simulink model "IEEE14_case"  (R2024b)
settings: Solver=FixedStepAuto  StartTime=0  StopTime=2  FixedStep=1e-7  RelTol=1e-3
values from neighbouring files (symbols this model uses):
  GFL_15_Bva = 0.009    [IEEE14_parameters.m]
  GFL_15_C_bus_pu = 7.179419    [IEEE14_parameters.m]
  GFL_15_f0 = 60    [IEEE14_parameters.m]
  GFL_15_I_id = 691.26967    [IEEE14_parameters.m]
  GFL_15_I_iq = 691.26967    [IEEE14_parameters.m]
  GFL_15_I_od = 45.2207    [IEEE14_parameters.m]
  GFL_15_I_oq = 45.2207    [IEEE14_parameters.m]
  GFL_15_I_pll = 0.78    [IEEE14_parameters.m]
  GFL_15_Kdi = 0.09    [IEEE14_parameters.m]
  GFL_15_Kdo = 0.9    [IEEE14_parameters.m]
  GFL_15_Kqi = 0.09    [IEEE14_parameters.m]
  GFL_15_Kqo = 0.9    [IEEE14_parameters.m]
  GFL_15_Lg_pu = 0.631447    [IEEE14_parameters.m]
  GFL_15_mode = 1    [IEEE14_parameters.m]
  GFL_15_P_id = 3.7166    [IEEE14_parameters.m]
  GFL_15_P_iq = 3.7166    [IEEE14_parameters.m]
  GFL_15_P_od = 0.4798    [IEEE14_parameters.m]
  GFL_15_P_oq = 0.4798    [IEEE14_parameters.m]
  GFL_15_P_pll = 290.42    [IEEE14_parameters.m]
  GFL_15_Qe_ref = 0.2    [IEEE14_parameters.m]
  GFL_15_Rg_pu = 0.024016    [IEEE14_parameters.m]
  GFL_15_Sbase = 1.000000e+4    (= 10000)    [IEEE14_parameters.m]
  GFL_15_Tdi = 0.01    [IEEE14_parameters.m]
  GFL_15_Tdo = 0.2    [IEEE14_parameters.m]
  GFL_15_Tqi = 0.01    [IEEE14_parameters.m]
  GFL_15_Tqo = 0.2    [IEEE14_parameters.m]
  GFL_15_Vbase = 380    [IEEE14_parameters.m]
  GFL_15_Vdc_ref = 1.011475    [IEEE14_parameters.m]
  GFL_15_Vdcbase = 700    [IEEE14_parameters.m]
  GFL_15_vq_ref = 0    [IEEE14_parameters.m]
  GFL_16_Bva = 0.002    [IEEE14_parameters.m]
  GFL_16_C_bus_pu = 7.179419    [IEEE14_parameters.m]
  GFL_16_f0 = 60    [IEEE14_parameters.m]
  GFL_16_I_id = 691.26967    [IEEE14_parameters.m]
  GFL_16_I_iq = 691.26967    [IEEE14_parameters.m]
  GFL_16_I_od = 45.2207    [IEEE14_parameters.m]
  GFL_16_I_oq = 45.2207    [IEEE14_parameters.m]
  GFL_16_I_pll = 0.78    [IEEE14_parameters.m]
  GFL_16_Kdi = 0.05    [IEEE14_parameters.m]
  GFL_16_Kdo = 0.5    [IEEE14_parameters.m]
  GFL_16_Kqi = 0.05    [IEEE14_parameters.m]
  GFL_16_Kqo = 0.5    [IEEE14_parameters.m]
  GFL_16_Lg_pu = 0.631447    [IEEE14_parameters.m]
  GFL_16_mode = 1    [IEEE14_parameters.m]
  GFL_16_P_id = 3.7166    [IEEE14_parameters.m]
  GFL_16_P_iq = 3.7166    [IEEE14_parameters.m]
  GFL_16_P_od = 0.4798    [IEEE14_parameters.m]
  GFL_16_P_oq = 0.4798    [IEEE14_parameters.m]
  GFL_16_P_pll = 290.42    [IEEE14_parameters.m]
  GFL_16_Qe_ref = 0.2    [IEEE14_parameters.m]
  GFL_16_Rg_pu = 0.024016    [IEEE14_parameters.m]
  GFL_16_Sbase = 1.000000e+4    (= 10000)    [IEEE14_parameters.m]
  GFL_16_Tdi = 0.01    [IEEE14_parameters.m]
  GFL_16_Tdo = 0.2    [IEEE14_parameters.m]
  GFL_16_Tqi = 0.01    [IEEE14_parameters.m]
  GFL_16_Tqo = 0.2    [IEEE14_parameters.m]
  GFL_16_Vbase = 380    [IEEE14_parameters.m]
  GFL_16_Vdc_ref = 1.01144    [IEEE14_parameters.m]
  GFL_16_Vdcbase = 700    [IEEE14_parameters.m]
  GFL_16_vq_ref = 0    [IEEE14_parameters.m]
  GFL_17_Bva = 0.002    [IEEE14_parameters.m]
  GFL_17_C_bus_pu = 7.179419    [IEEE14_parameters.m]
  GFL_17_f0 = 60    [IEEE14_parameters.m]
  GFL_17_I_id = 691.26967    [IEEE14_parameters.m]
  GFL_17_I_iq = 691.26967    [IEEE14_parameters.m]
  GFL_17_I_od = 45.2207    [IEEE14_parameters.m]
  GFL_17_I_oq = 45.2207    [IEEE14_parameters.m]
  GFL_17_I_pll = 0.78    [IEEE14_parameters.m]
  GFL_17_Kdi = 0.05    [IEEE14_parameters.m]
  GFL_17_Kdo = 0.5    [IEEE14_parameters.m]
  GFL_17_Kqi = 0.05    [IEEE14_parameters.m]
  GFL_17_Kqo = 0.5    [IEEE14_parameters.m]
  GFL_17_Lg_pu = 0.631447    [IEEE14_parameters.m]
  GFL_17_mode = 1    [IEEE14_parameters.m]
  GFL_17_P_id = 3.7166    [IEEE14_parameters.m]
  GFL_17_P_iq = 3.7166    [IEEE14_parameters.m]
  GFL_17_P_od = 0.4798    [IEEE14_parameters.m]
  GFL_17_P_oq = 0.4798    [IEEE14_parameters.m]
  GFL_17_P_pll = 290.42    [IEEE14_parameters.m]
  GFL_17_Qe_ref = 0.2    [IEEE14_parameters.m]
  GFL_17_Rg_pu = 0.024016    [IEEE14_parameters.m]
  GFL_17_Sbase = 1.000000e+4    (= 10000)    [IEEE14_parameters.m]
  GFL_17_Tdi = 0.01    [IEEE14_parameters.m]
  GFL_17_Tdo = 0.2    [IEEE14_parameters.m]
  GFL_17_Tqi = 0.01    [IEEE14_parameters.m]
  GFL_17_Tqo = 0.2    [IEEE14_parameters.m]
  GFL_17_Vbase = 380    [IEEE14_parameters.m]
  GFL_17_Vdc_ref = 1.011632    [IEEE14_parameters.m]
  GFL_17_Vdcbase = 700    [IEEE14_parameters.m]
  GFL_17_vq_ref = 0    [IEEE14_parameters.m]
  GFL_18_Bva = 0.002    [IEEE14_parameters.m]
  GFL_18_C_bus_pu = 7.179419    [IEEE14_parameters.m]
  GFL_18_f0 = 60    [IEEE14_parameters.m]
  GFL_18_I_id = 691.26967    [IEEE14_parameters.m]
  GFL_18_I_iq = 691.26967    [IEEE14_parameters.m]
  GFL_18_I_od = 45.2207    [IEEE14_parameters.m]
  GFL_18_I_oq = 45.2207    [IEEE14_parameters.m]
  GFL_18_I_pll = 0.78    [IEEE14_parameters.m]
  GFL_18_Kdi = 0.05    [IEEE14_parameters.m]
  GFL_18_Kdo = 0.5    [IEEE14_parameters.m]
  GFL_18_Kqi = 0.05    [IEEE14_parameters.m]
  GFL_18_Kqo = 0.5    [IEEE14_parameters.m]
  GFL_18_Lg_pu = 0.631447    [IEEE14_parameters.m]
  GFL_18_mode = 1    [IEEE14_parameters.m]
  GFL_18_P_id = 3.7166    [IEEE14_parameters.m]
  GFL_18_P_iq = 3.7166    [IEEE14_parameters.m]
  GFL_18_P_od = 0.4798    [IEEE14_parameters.m]
  GFL_18_P_oq = 0.4798    [IEEE14_parameters.m]
  GFL_18_P_pll = 290.42    [IEEE14_parameters.m]
  GFL_18_Qe_ref = 0.2    [IEEE14_parameters.m]
  GFL_18_Rg_pu = 0.024016    [IEEE14_parameters.m]
  GFL_18_Sbase = 1.000000e+4    (= 10000)    [IEEE14_parameters.m]
  GFL_18_Tdi = 0.01    [IEEE14_parameters.m]
  GFL_18_Tdo = 0.2    [IEEE14_parameters.m]
  GFL_18_Tqi = 0.01    [IEEE14_parameters.m]
  GFL_18_Tqo = 0.2    [IEEE14_parameters.m]
  GFL_18_Vbase = 380    [IEEE14_parameters.m]
  GFL_18_Vdc_ref = 1.011572    [IEEE14_parameters.m]
  GFL_18_Vdcbase = 700    [IEEE14_parameters.m]
  GFL_18_vq_ref = 0    [IEEE14_parameters.m]
  ... (+180 more)
(part 10 of 25)

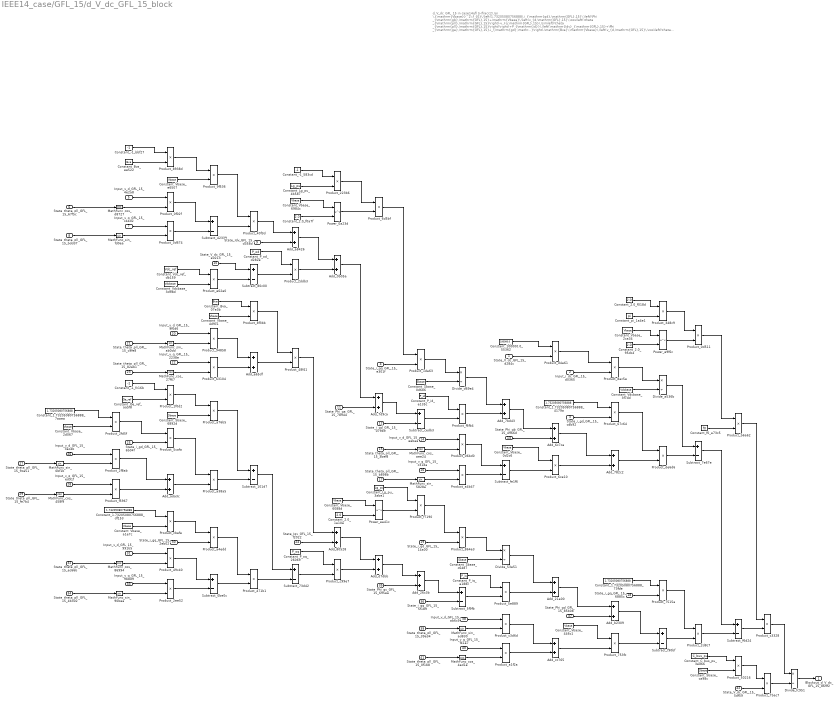
== system IEEE14_case/GFL_15/d_V_dc_GFL_15_block ==
  note: d_V_dc_GFL_15 in case14gfl
      | $-\frac{2\,\pi \,{\mathrm{Vbase}}^2\,f_{0}\,\left(1.73205080756888\,i_{\mathrm{gd},\mathrm{GFL},15}\,\left(\Phi _{\mathrm{gb},\mathrm{GFL},15}+\mathrm{Vbase}\,\left(v_{d,\mathrm{GFL},15}\,\cos\left(\theta _{\mathrm{pll},\mathrm{GFL},15}\right)-v_{q,\mathrm{GFL},15}\,\sin\left(\theta _{\mathrm{pll},\mathrm{GFL},15}\right)\right)+P_{\mathrm{id}}\,\left(\mathrm{Idv}_{\mathrm{GFL},15}+\Phi _{\mathrm{ga},\mathrm{GFL},15}-i_{\mathrm{gd},\mathrm{GFL},15}+P_{\mathrm{od}}\,\left(V_{\mathrm{dc},\mathrm{GFL},15}-\mathrm{Vdcbase}\,\mathrm{Vdc}_{\mathrm{ref}}\right)-\mathrm{Bva}\,\mathrm{Vbase}\,\left(v_{d,\mathrm{GFL},15}\,\cos\left(\theta _{\mathrm{pll},\mathrm{GFL},15}\right)-v_{q,\mathrm{GFL},15}\,\sin\left(\theta _{\mathrm{pll},\mathrm{GFL},15}\right)\right)\right)-\frac{\mathrm{Lg}_{\mathrm{pu}}\,{\mathrm{Vbase}}^2\,i_{\mathrm{gq},\mathrm{GFL},15}}{\mathrm{Sbase}}\right)+1.73205080756888\,i_{\mathrm{gq},\mathrm{GFL},15}\,\left(\Phi _{\mathrm{gd},\mathrm{GFL},15}-\mathrm{Vbase}\,\left(v_{q,\mathrm{GFL},15}\,\cos\left(\theta _{\mathrm{pll},\mathrm{GFL},15}\right)+v_{d,\mathrm{GFL},15}\,\sin\left(\theta _{\mathrm{pll},\mathrm{GFL},15}\right)\right)+P_{\mathrm{iq}}\,\left(\mathrm{Iqv}_{\mathrm{GFL},15}+\Phi _{\mathrm{gc},\mathrm{GFL},15}-i_{\mathrm{gq},\mathrm{GFL},15}-P_{\mathrm{oq}}\,\left(\mathrm{Qe}_{\mathrm{ref}}\,\mathrm{Sbase}+1.73205080756888\,\mathrm{Vbase}\,i_{\mathrm{gd},\mathrm{GFL},15}\,\left(v_{q,\mathrm{GFL},15}\,\cos\left(\theta _{\mathrm{pll},\mathrm{GFL},15}\right)+v_{d,\mathrm{GFL},15}\,\sin\left(\theta _{\mathrm{pll},\mathrm{GFL},15}\right)\right)+1.73205080756888\,\mathrm{Vbase}\,i_{\mathrm{gq},\mathrm{GFL},15}\,\left(v_{d,\mathrm{GFL},15}\,\cos\left(\theta _{\mathrm{pll},\mathrm{GFL},15}\right)-v_{q,\mathrm{GFL},15}\,\sin\left(\theta _{\mathrm{pll},\mathrm{GFL},15}\right)\right)\right)+\mathrm{Bva}\,\mathrm{Vbase}\,\left(v_{q,\mathrm{GFL},15}\,\cos\left(\theta _{\mathrm{pll},\mathrm{GFL},15}\right)+v_{d,\mathrm{GFL},15}\,\sin\left(\theta _{\mathrm{pll},\mathrm{GFL},15}\right)\right)\right)+\frac{\mathrm{Lg}_{\mathrm{pu}}\,{\mathrm{Vbase}}^2\,i_{\mathrm{gd},\mathrm{GFL},15}}{\mathrm{Sbase}}\right)-\frac{100000.0\,V_{\mathrm{dc},\mathrm{GFL},15}\,i_{\mathrm{dc},\mathrm{GFL},15}}{\mathrm{Vdcbase}}\right)}{C_{\mathrm{bus},\mathrm{pu}}\,\mathrm{Sbase}\,V_{\mathrm{dc},\mathrm{GFL},15}}$
      | Automatically generated on 2025-10-09 21:35:09 .
  State_V_dc_GFL_15_d284c : Inport
  Input_i_dc_GFL_15_d0365 : Inport  Port=2
  State_i_gd_GFL_15_cdb92 : Inport  Port=3
  State_i_gq_GFL_15_e301f : Inport  Port=4
  Input_v_d_GFL_15_4e2a8 : Inport  Port=5
  State_theta_pll_GFL_15_67f5c : Inport  Port=6
  Input_v_q_GFL_15_c44d2 : Inport  Port=7
  State_theta_pll_GFL_15_bdd37 : Inport  Port=8
  State_Idv_GFL_15_d358d : Inport  Port=9
  State_V_dc_GFL_15_e0213 : Inport  Port=10
  State_Phi_ga_GFL_15_78944 : Inport  Port=11
  State_i_gd_GFL_15_079b9 : Inport  Port=12
  State_Phi_gb_GFL_15_4966d : Inport  Port=13
  Input_v_d_GFL_15_eebae : Inport  Port=14
  State_theta_pll_GFL_15_3bef8 : Inport  Port=15
  Input_v_q_GFL_15_c31da : Inport  Port=16
  State_theta_pll_GFL_15_b898b : Inport  Port=17
  State_i_gq_GFL_15_6885c : Inport  Port=18
  State_i_gd_GFL_15_14a00 : Inport  Port=19
  Input_v_d_GFL_15_9f0d6 : Inport  Port=20
  State_theta_pll_GFL_15_c9fe8 : Inport  Port=21
  Input_v_q_GFL_15_2238e : Inport  Port=22
  State_theta_pll_GFL_15_82eb1 : Inport  Port=23
  State_Iqv_GFL_15_f2022 : Inport  Port=24
  State_i_gd_GFL_15_6b04f : Inport  Port=25
  Input_v_d_GFL_15_3ac4b : Inport  Port=26
  State_theta_pll_GFL_15_9ca51 : Inport  Port=27
  Input_v_q_GFL_15_ed91f : Inport  Port=28
  State_theta_pll_GFL_15_fe7b4 : Inport  Port=29
  State_i_gq_GFL_15_2eb02 : Inport  Port=30
  Input_v_d_GFL_15_991b5 : Inport  Port=31
  State_theta_pll_GFL_15_ec66b : Inport  Port=32
  Input_v_q_GFL_15_9b8d9 : Inport  Port=33
  State_theta_pll_GFL_15_4b302 : Inport  Port=34
  State_Phi_gc_GFL_15_695ea : Inport  Port=35
  State_i_gq_GFL_15_5f189 : Inport  Port=36
  State_Phi_gd_GFL_15_85b08 : Inport  Port=37
  Input_v_d_GFL_15_ab6c9 : Inport  Port=38
  State_theta_pll_GFL_15_39e34 : Inport  Port=39
  Input_v_q_GFL_15_f41a7 : Inport  Port=40
  State_theta_pll_GFL_15_0f1b8 : Inport  Port=41
  State_V_dc_GFL_15_5df59 : Inport  Port=42
  Add_0b05a : Sum
  Add_21a00 : Sum
  Add_26c3b : Sum
  Add_6c7ca : Sum
  Add_782c2 : Sum
  Add_7bd43 : Sum
  Add_7d9ca : Sum
  Add_80528 : Sum
  Add_a8426 : Sum
  Add_ada3c : Sum
  Add_b2309 : Sum
  Add_cc765 : Sum
  Add_d7dbb : Sum
  Add_e65df : Sum
  Constant_-1_583cd : Constant  Value=-1
  Constant_-1_bbf27 : Constant  Value=-1
  Constant_-1_fc16b : Constant  Value=-1
  Constant_1.73205080756888_4179a : Constant  Value=1.73205080756888
  Constant_1.73205080756888_73fde : Constant  Value=1.73205080756888
  Constant_1.73205080756888_7aaea : Constant  Value=1.73205080756888
  Constant_1.73205080756888_df153 : Constant  Value=1.73205080756888
  Constant_100000.0_55362 : Constant  Value=100000.0
  Constant_2.0_1a10a : Constant  Value=2.0
  Constant_2.0_95cb4 : Constant  Value=2.0
  Constant_2.0_f018d : Constant  Value=2.0
  Constant_2.0_f0a7f : Constant  Value=2.0
  Constant_Bva_07e3b : Constant  Value=Bva
  Constant_Bva_ee522 : Constant  Value=Bva
  Constant_C_bus_pu_3ed66 : Constant  Value=C_bus_pu
  Constant_Lg_pu_3abe1 : Constant  Value=Lg_pu
  Constant_Lg_pu_4b587 : Constant  Value=Lg_pu
  Constant_P_id_e135c : Constant  Value=P_id
  Constant_P_iq_a188c : Constant  Value=P_iq
  Constant_P_od_d282e : Constant  Value=P_od
  Constant_P_oq_26069 : Constant  Value=P_oq
  Constant_Qe_ref_aa5f8 : Constant  Value=Qe_ref
  Constant_Sbase_0d6b6 : Constant  Value=Sbase
  Constant_Sbase_6892d : Constant  Value=Sbase
  Constant_Sbase_c6487 : Constant  Value=Sbase
  Constant_Sbase_ca98c : Constant  Value=Sbase
  Constant_Vbase_0d2c6 : Constant  Value=Vbase
  Constant_Vbase_2ca34 : Constant  Value=Vbase
  Constant_Vbase_2d067 : Constant  Value=Vbase
  Constant_Vbase_446c1 : Constant  Value=Vbase
  Constant_Vbase_4d9c1 : Constant  Value=Vbase
  Constant_Vbase_6088d : Constant  Value=Vbase
  Constant_Vbase_6984c : Constant  Value=Vbase
  Constant_Vbase_a1e7c : Constant  Value=Vbase
  Constant_Vbase_e6507 : Constant  Value=Vbase
  Constant_Vdc_ref_db159 : Constant  Value=Vdc_ref
  Constant_Vdcbase_3d98d : Constant  Value=Vdcbase
  Constant_Vdcbase_3f7dd : Constant  Value=Vdcbase
  Constant_f0_a73c5 : Constant  Value=f0
  Constant_pi_1a4e1 : Constant  Value=pi
  Divide_53e51 : Product  Inputs=*/
  Divide_a536b : Product  Inputs=*/
  Divide_d69e4 : Product  Inputs=*/
  Divide_fc951 : Product  Inputs=*/
  MathFunc_cos_27f67 : Trigonometry  Operator=cos
  MathFunc_cos_458f9 : Trigonometry  Operator=cos
  MathFunc_cos_4ad1e : Trigonometry  Operator=cos
  MathFunc_cos_86994 : Trigonometry  Operator=cos
  MathFunc_cos_aee24 : Trigonometry  Operator=cos
  MathFunc_cos_d8727 : Trigonometry  Operator=cos
  MathFunc_sin_0bf1b : Trigonometry
  MathFunc_sin_5828a : Trigonometry
  MathFunc_sin_90bea : Trigonometry
  MathFunc_sin_ab0dd : Trigonometry
  MathFunc_sin_ad830 : Trigonometry
  MathFunc_sin_fd0ea : Trigonometry
  Power_0a23d : Math  Operator=pow
  Power_e9f6c : Math  Operator=pow
  Power_ea41c : Math  Operator=pow
  Product_06bd0 : Product
  Product_0d511 : Product
  Product_0f02f : Product
  Product_1da63 : Product
  Product_1f0d2 : Product
  Product_223b6 : Product
  Product_2d8c7 : Product
  Product_2ddb3 : Product
  Product_2ee52 : Product
  Product_2f8ab : Product
  Product_2fd5f : Product
  Product_348c9 : Product
  Product_3d674 : Product
  Product_40f3d : Product
  Product_471b1 : Product
  Product_48f41 : Product
  Product_49c40 : Product
  Product_50216 : Product
  Product_5cafa : Product
  Product_5e889 : Product
  Product_63104 : Product
  Product_67c64 : Product
  Product_6ce10 : Product
  Product_6d5bf : Product
  Product_7515a : Product
  Product_753fc : Product
  Product_7bac7 : Product
  Product_864e3 : Product
  Product_8938d : Product
  Product_8ac5e : Product
  Product_8f3bb : Product
  Product_94858 : Product
  Product_9f536 : Product
  Product_a1f2a : Product
  Product_a38a5 : Product
  Product_a4b47 : Product
  Product_a4edd : Product
  Product_a76b5 : Product
  Product_b6a62 : Product
  Product_c3328 : Product
  Product_c3d6d : Product
  Product_c99e7 : Product
  Product_cbefe : Product
  Product_d4a61 : Product
  Product_de6d6 : Product
  Product_e62e0 : Product
  Product_f5967 : Product
  Product_f6fb4 : Product
  Product_f7190 : Product
  Subtract_0be0c : Sum  Inputs=+-
  Subtract_101d7 : Sum  Inputs=+-
  Subtract_42339 : Sum  Inputs=+-
  Subtract_5f9fb : Sum  Inputs=+-
  Subtract_73d42 : Sum  Inputs=+-
  Subtract_7e67e : Sum  Inputs=+-
  Subtract_80c00 : Sum  Inputs=+-
  Subtract_cedb3 : Sum  Inputs=+-
  Subtract_f6d24 : Sum  Inputs=+-
  Subtract_f90bf : Sum  Inputs=+-
  Subtract_fe1f6 : Sum  Inputs=+-
  Blockout_d_V_dc_GFL_15_869f2 : Outport
  wires:
  Product_cbefe/1 -> Product_a4edd/1
  State_Phi_gd_GFL_15_85b08/1 -> Add_b2309/2
  Subtract_f6d24/1 -> Product_c3328/2
  State_i_gd_GFL_15_6b04f/1 -> Product_5cafa/2
  Product_7bac7/1 -> Divide_fc951/2
  State_V_dc_GFL_15_d284c/1 -> Product_d4a61/2
  State_theta_pll_GFL_15_b898b/1 -> MathFunc_sin_5828a/1
  Product_2fd5f/1 -> Product_5cafa/1
  Constant_Sbase_ca98c/1 -> Product_50216/2
  Divide_fc951/1 -> Blockout_d_V_dc_GFL_15_869f2/1
  Product_50216/1 -> Product_7bac7/1
  Input_v_d_GFL_15_991b5/1 -> Product_49c40/1
  State_Idv_GFL_15_d358d/1 -> Add_a8426/2
  Subtract_73d42/1 -> Product_c99e7/2
  Constant_-1_fc16b/1 -> Product_1f0d2/1
  Product_2d8c7/1 -> Subtract_f6d24/2
  Add_21a00/1 -> Add_b2309/1
  Product_d4a61/1 -> Product_8ac5e/1
  Product_348c9/1 -> Product_0d511/1
  Add_cc765/1 -> Product_753fc/2
  State_V_dc_GFL_15_5df59/1 -> Product_7bac7/2
  Product_7515a/1 -> Product_2d8c7/1
  Constant_C_bus_pu_3ed66/1 -> Product_50216/1
  Subtract_101d7/1 -> Subtract_73d42/1
  Product_c3328/1 -> Divide_fc951/1
  State_theta_pll_GFL_15_9ca51/1 -> MathFunc_sin_0bf1b/1
  Input_v_d_GFL_15_ab6c9/1 -> Product_c3d6d/1
  Subtract_f90bf/1 -> Product_2d8c7/2
  Product_6d5bf/1 -> Product_1da63/1
  Product_753fc/1 -> Subtract_f90bf/2
  Product_2ee52/1 -> Subtract_0be0c/2
  Input_v_q_GFL_15_9b8d9/1 -> Product_2ee52/1
  Add_26c3b/1 -> Subtract_5f9fb/1
  Product_5cafa/1 -> Product_a38a5/1
  MathFunc_sin_5828a/1 -> Product_a4b47/2
  Add_e65df/1 -> Product_48f41/2
  Subtract_0be0c/1 -> Product_471b1/2
  Subtract_7e67e/1 -> Subtract_f6d24/1
  State_theta_pll_GFL_15_39e34/1 -> MathFunc_sin_ad830/1
  Add_b2309/1 -> Subtract_f90bf/1
  MathFunc_sin_ad830/1 -> Product_c3d6d/2
  Product_a1f2a/1 -> Add_cc765/2
  MathFunc_cos_4ad1e/1 -> Product_a1f2a/2
  State_theta_pll_GFL_15_0f1b8/1 -> MathFunc_cos_4ad1e/1
  Input_v_q_GFL_15_f41a7/1 -> Product_a1f2a/1
  Product_5e889/1 -> Add_21a00/2
  Input_v_q_GFL_15_c44d2/1 -> Product_3d674/1
  Product_f5967/1 -> Add_ada3c/2
  State_theta_pll_GFL_15_ec66b/1 -> MathFunc_cos_86994/1
  Product_c3d6d/1 -> Add_cc765/1
  Product_a38a5/1 -> Subtract_101d7/2
  State_i_gq_GFL_15_2eb02/1 -> Product_a4edd/2
  Product_f7190/1 -> Product_864e3/1
  Constant_Vbase_446c1/1 -> Product_753fc/1
  State_i_gq_GFL_15_5f189/1 -> Subtract_5f9fb/2
  Subtract_5f9fb/1 -> Product_5e889/2
  Add_ada3c/1 -> Product_a38a5/2
  State_Phi_gc_GFL_15_695ea/1 -> Add_26c3b/2
  Add_d7dbb/1 -> Add_26c3b/1
  MathFunc_cos_86994/1 -> Product_49c40/2
  Product_c99e7/1 -> Add_d7dbb/2
  Input_v_d_GFL_15_3ac4b/1 -> Product_2f8ab/1
  Product_471b1/1 -> Subtract_73d42/2
  Product_6ce10/1 -> Add_782c2/2
  Product_1f0d2/1 -> Product_a76b5/1
  Constant_2.0_1a10a/1 -> Power_ea41c/2
  Constant_Vbase_2d067/1 -> Product_2fd5f/2
  Product_49c40/1 -> Subtract_0be0c/1
  MathFunc_cos_27f67/1 -> Product_63104/2
  MathFunc_sin_90bea/1 -> Product_2ee52/2
  State_theta_pll_GFL_15_4b302/1 -> MathFunc_sin_90bea/1
  State_theta_pll_GFL_15_82eb1/1 -> MathFunc_cos_27f67/1
  Product_a4edd/1 -> Product_471b1/1
  Constant_1.73205080756888_7aaea/1 -> Product_2fd5f/1
  Subtract_42339/1 -> Product_40f3d/2
  Constant_Vbase_a1e7c/1 -> Product_cbefe/2
  Constant_1.73205080756888_df153/1 -> Product_cbefe/1
  MathFunc_cos_458f9/1 -> Product_f5967/2
  State_theta_pll_GFL_15_fe7b4/1 -> MathFunc_cos_458f9/1
  Input_v_q_GFL_15_ed91f/1 -> Product_f5967/1
  Product_2f8ab/1 -> Add_ada3c/1
  MathFunc_sin_0bf1b/1 -> Product_2f8ab/2
  Product_f6fb4/1 -> Add_7bd43/2
  Product_a76b5/1 -> Subtract_101d7/1
  Constant_Sbase_6892d/1 -> Product_a76b5/2
  Constant_Qe_ref_aa5f8/1 -> Product_1f0d2/2
  Product_0d511/1 -> Product_b6a62/1
  Input_v_d_GFL_15_eebae/1 -> Product_06bd0/1
  Constant_P_oq_26069/1 -> Product_c99e7/1
  Add_80528/1 -> Add_d7dbb/1
  State_Iqv_GFL_15_f2022/1 -> Add_80528/2
  Product_48f41/1 -> Add_80528/1
  Constant_Vdcbase_3f7dd/1 -> Divide_a536b/2
  Product_63104/1 -> Add_e65df/2
  Input_v_q_GFL_15_2238e/1 -> Product_63104/1
  Product_94858/1 -> Add_e65df/1
  Product_8ac5e/1 -> Divide_a536b/1
  MathFunc_sin_ab0dd/1 -> Product_94858/2
  State_theta_pll_GFL_15_c9fe8/1 -> MathFunc_sin_ab0dd/1
  Input_v_d_GFL_15_9f0d6/1 -> Product_94858/1
  Product_8f3bb/1 -> Product_48f41/1
  Product_9f536/1 -> Product_40f3d/1
  Constant_Vbase_4d9c1/1 -> Product_8f3bb/2
  State_theta_pll_GFL_15_bdd37/1 -> MathFunc_sin_fd0ea/1
  Constant_Bva_07e3b/1 -> Product_8f3bb/1
  Subtract_80c00/1 -> Product_2ddb3/2
  Constant_P_iq_a188c/1 -> Product_5e889/1
  Divide_53e51/1 -> Add_21a00/1
  Constant_Sbase_c6487/1 -> Divide_53e51/2
  Product_864e3/1 -> Divide_53e51/1
  State_i_gd_GFL_15_14a00/1 -> Product_864e3/2
  Power_ea41c/1 -> Product_f7190/2
  Constant_1.73205080756888_4179a/1 -> Product_67c64/1
  Constant_Vbase_6088d/1 -> Power_ea41c/1
  Constant_Lg_pu_3abe1/1 -> Product_f7190/1
  State_i_gq_GFL_15_6885c/1 -> Product_7515a/2
  Constant_1.73205080756888_73fde/1 -> Product_7515a/1
  Product_de6d6/1 -> Subtract_7e67e/2
  Constant_-1_583cd/1 -> Product_223b6/1
  Constant_P_id_e135c/1 -> Product_f6fb4/1
  Add_782c2/1 -> Product_de6d6/2
  State_Phi_gb_GFL_15_4966d/1 -> Add_6c7ca/2
  Constant_Lg_pu_4b587/1 -> Product_223b6/2
  Add_7d9ca/1 -> Subtract_cedb3/1
  Subtract_fe1f6/1 -> Product_6ce10/2
  Product_a4b47/1 -> Subtract_fe1f6/2
  Input_v_q_GFL_15_c31da/1 -> Product_a4b47/1
  Product_06bd0/1 -> Subtract_fe1f6/1
  MathFunc_cos_aee24/1 -> Product_06bd0/2
  State_theta_pll_GFL_15_3bef8/1 -> MathFunc_cos_aee24/1
  Constant_Vbase_6984c/1 -> Power_0a23d/1
  Constant_Vbase_0d2c6/1 -> Product_6ce10/1
  Add_6c7ca/1 -> Add_782c2/1
  Add_7bd43/1 -> Add_6c7ca/1
  Subtract_cedb3/1 -> Product_f6fb4/2
  State_i_gd_GFL_15_079b9/1 -> Subtract_cedb3/2
  State_Phi_ga_GFL_15_78944/1 -> Add_7d9ca/2
  Add_0b05a/1 -> Add_7d9ca/1
  Product_2ddb3/1 -> Add_0b05a/2
  Product_e62e0/1 -> Subtract_80c00/2
  Constant_Vdcbase_3d98d/1 -> Product_e62e0/2
  Constant_Vdc_ref_db159/1 -> Product_e62e0/1
  Product_1da63/1 -> Divide_d69e4/1
  State_V_dc_GFL_15_e0213/1 -> Subtract_80c00/1
  Constant_P_od_d282e/1 -> Product_2ddb3/1
  Add_a8426/1 -> Add_0b05a/1
  Product_40f3d/1 -> Add_a8426/1
  Constant_Vbase_2ca34/1 -> Power_e9f6c/1
  Product_3d674/1 -> Subtract_42339/2
  MathFunc_sin_fd0ea/1 -> Product_3d674/2
  Product_0f02f/1 -> Subtract_42339/1
  MathFunc_cos_d8727/1 -> Product_0f02f/2
  State_theta_pll_GFL_15_67f5c/1 -> MathFunc_cos_d8727/1
  Input_v_d_GFL_15_4e2a8/1 -> Product_0f02f/1
  Constant_Vbase_e6507/1 -> Product_9f536/2
  Product_8938d/1 -> Product_9f536/1
  Constant_Bva_ee522/1 -> Product_8938d/2
  Constant_-1_bbf27/1 -> Product_8938d/1
  Divide_d69e4/1 -> Add_7bd43/1
  Constant_Sbase_0d6b6/1 -> Divide_d69e4/2
  State_i_gq_GFL_15_e301f/1 -> Product_1da63/2
  Power_0a23d/1 -> Product_6d5bf/2
  Constant_2.0_f0a7f/1 -> Power_0a23d/2
  Product_223b6/1 -> Product_6d5bf/1
  Input_i_dc_GFL_15_d0365/1 -> Product_8ac5e/2
  Product_67c64/1 -> Product_de6d6/1
  State_i_gd_GFL_15_cdb92/1 -> Product_67c64/2
  Divide_a536b/1 -> Subtract_7e67e/1
  Constant_100000.0_55362/1 -> Product_d4a61/1
  Product_b6a62/1 -> Product_c3328/1
  Constant_f0_a73c5/1 -> Product_b6a62/2
  Power_e9f6c/1 -> Product_0d511/2
  Constant_2.0_95cb4/1 -> Power_e9f6c/2
  Constant_pi_1a4e1/1 -> Product_348c9/2
  Constant_2.0_f018d/1 -> Product_348c9/1

== system IEEE14_case/GFL_15/d_i_gd_GFL_15_block ==
  note: d_i_gd_GFL_15 in case14gfl
      | $\frac{2\,\pi \,\mathrm{Sbase}\,f_{0}\,\left(\Phi _{\mathrm{gb},\mathrm{GFL},15}+P_{\mathrm{id}}\,\left(\mathrm{Idv}_{\mathrm{GFL},15}+\Phi _{\mathrm{ga},\mathrm{GFL},15}-i_{\mathrm{gd},\mathrm{GFL},15}+P_{\mathrm{od}}\,\left(V_{\mathrm{dc},\mathrm{GFL},15}-\mathrm{Vdcbase}\,\mathrm{Vdc}_{\mathrm{ref}}\right)-\mathrm{Bva}\,\mathrm{Vbase}\,\left(v_{d,\mathrm{GFL},15}\,\cos\left(\theta _{\mathrm{pll},\mathrm{GFL},15}\right)-v_{q,\mathrm{GFL},15}\,\sin\left(\theta _{\mathrm{pll},\mathrm{GFL},15}\right)\right)\right)-\frac{\mathrm{Rg}_{\mathrm{pu}}\,{\mathrm{Vbase}}^2\,i_{\mathrm{gd},\mathrm{GFL},15}}{\mathrm{Sbase}}\right)}{\mathrm{Lg}_{\mathrm{pu}}\,{\mathrm{Vbase}}^2}$
      | Automatically generated on 2025-10-09 21:34:51 .
  Input_v_d_GFL_15_1fa3a : Inport
  State_theta_pll_GFL_15_a07ec : Inport  Port=2
  Input_v_q_GFL_15_bfddf : Inport  Port=3
  State_theta_pll_GFL_15_781ce : Inport  Port=4
  State_Idv_GFL_15_0b38b : Inport  Port=5
  State_V_dc_GFL_15_5ead9 : Inport  Port=6
  State_Phi_ga_GFL_15_6d748 : Inport  Port=7
  State_i_gd_GFL_15_d802d : Inport  Port=8
  State_Phi_gb_GFL_15_ef282 : Inport  Port=9
  State_i_gd_GFL_15_48775 : Inport  Port=10
  Add_1112d : Sum
  Add_483a0 : Sum
  Add_a0179 : Sum
  Add_cadd7 : Sum
  Constant_-1_8e1f0 : Constant  Value=-1
  Constant_2.0_01abc : Constant  Value=2.0
  Constant_2.0_5bfd0 : Constant  Value=2.0
  Constant_2.0_e9fc9 : Constant  Value=2.0
  Constant_Bva_be5e7 : Constant  Value=Bva
  Constant_Lg_pu_53032 : Constant  Value=Lg_pu
  Constant_P_id_a7916 : Constant  Value=P_id
  Constant_P_od_047fb : Constant  Value=P_od
  Constant_Rg_pu_4475c : Constant  Value=Rg_pu
  Constant_Sbase_2e4f4 : Constant  Value=Sbase
  Constant_Sbase_a3e46 : Constant  Value=Sbase
  Constant_Vbase_0c6e1 : Constant  Value=Vbase
  Constant_Vbase_4a526 : Constant  Value=Vbase
  Constant_Vbase_f32af : Constant  Value=Vbase
  Constant_Vdc_ref_11b54 : Constant  Value=Vdc_ref
  Constant_Vdcbase_f3ba6 : Constant  Value=Vdcbase
  Constant_f0_04d95 : Constant  Value=f0
  Constant_pi_78564 : Constant  Value=pi
  Divide_0427d : Product  Inputs=*/
  Divide_fbc70 : Product  Inputs=*/
  MathFunc_cos_b3ca8 : Trigonometry  Operator=cos
  MathFunc_sin_00092 : Trigonometry
  Power_4da07 : Math  Operator=pow
  Power_5170c : Math  Operator=pow
  Product_14e40 : Product
  Product_2bdaa : Product
  Product_419c8 : Product
  Product_5b870 : Product
  Product_5bc1d : Product
  Product_68778 : Product
  Product_6b2f9 : Product
  Product_8930e : Product
  Product_aa72d : Product
  Product_ba359 : Product
  Product_cc95f : Product
  Product_cea5c : Product
  Product_e5499 : Product
  Product_ea684 : Product
  Product_f6633 : Product
  Subtract_06b24 : Sum  Inputs=+-
  Subtract_61ff1 : Sum  Inputs=+-
  Subtract_9f9a0 : Sum  Inputs=+-
  Subtract_e16d7 : Sum  Inputs=+-
  Blockout_d_i_gd_GFL_15_2c157 : Outport
  wires:
  State_theta_pll_GFL_15_a07ec/1 -> MathFunc_cos_b3ca8/1
  State_theta_pll_GFL_15_781ce/1 -> MathFunc_sin_00092/1
  MathFunc_sin_00092/1 -> Product_cea5c/2
  Product_aa72d/1 -> Subtract_9f9a0/2
  Constant_Vdc_ref_11b54/1 -> Product_aa72d/1
  Constant_Bva_be5e7/1 -> Product_cc95f/2
  Product_cc95f/1 -> Product_68778/1
  Constant_-1_8e1f0/1 -> Product_cc95f/1
  Product_14e40/1 -> Subtract_06b24/1
  Input_v_d_GFL_15_1fa3a/1 -> Product_14e40/1
  MathFunc_cos_b3ca8/1 -> Product_14e40/2
  Product_cea5c/1 -> Subtract_06b24/2
  Input_v_q_GFL_15_bfddf/1 -> Product_cea5c/1
  Constant_Vbase_0c6e1/1 -> Product_68778/2
  Product_e5499/1 -> Add_483a0/1
  Constant_Vdcbase_f3ba6/1 -> Product_aa72d/2
  Product_68778/1 -> Product_e5499/1
  Subtract_06b24/1 -> Product_e5499/2
  Subtract_9f9a0/1 -> Product_f6633/2
  State_V_dc_GFL_15_5ead9/1 -> Subtract_9f9a0/1
  State_Idv_GFL_15_0b38b/1 -> Add_483a0/2
  Product_f6633/1 -> Add_a0179/2
  Constant_P_od_047fb/1 -> Product_f6633/1
  Add_483a0/1 -> Add_a0179/1
  Add_a0179/1 -> Add_cadd7/1
  State_Phi_ga_GFL_15_6d748/1 -> Add_cadd7/2
  Constant_Sbase_2e4f4/1 -> Product_6b2f9/2
  Power_4da07/1 -> Product_419c8/2
  Constant_Vbase_f32af/1 -> Power_4da07/1
  Constant_f0_04d95/1 -> Product_8930e/2
  Constant_2.0_e9fc9/1 -> Power_4da07/2
  Add_cadd7/1 -> Subtract_e16d7/1
  State_i_gd_GFL_15_d802d/1 -> Subtract_e16d7/2
  Constant_Rg_pu_4475c/1 -> Product_419c8/1
  State_i_gd_GFL_15_48775/1 -> Product_5b870/2
  Constant_2.0_5bfd0/1 -> Product_ea684/1
  Constant_pi_78564/1 -> Product_ea684/2
  Constant_P_id_a7916/1 -> Product_5bc1d/1
  Subtract_e16d7/1 -> Product_5bc1d/2
  Product_419c8/1 -> Product_5b870/1
  Product_ea684/1 -> Product_6b2f9/1
  Product_5bc1d/1 -> Add_1112d/1
  State_Phi_gb_GFL_15_ef282/1 -> Add_1112d/2
  Product_5b870/1 -> Divide_fbc70/1
  Product_6b2f9/1 -> Product_8930e/1
  Constant_Sbase_a3e46/1 -> Divide_fbc70/2
  Add_1112d/1 -> Subtract_61ff1/1
  Divide_fbc70/1 -> Subtract_61ff1/2
  Constant_2.0_01abc/1 -> Power_5170c/2
  Constant_Vbase_4a526/1 -> Power_5170c/1
  Product_8930e/1 -> Product_ba359/1
  Subtract_61ff1/1 -> Product_ba359/2
  Product_2bdaa/1 -> Divide_0427d/2
  Constant_Lg_pu_53032/1 -> Product_2bdaa/1
  Power_5170c/1 -> Product_2bdaa/2
  Product_ba359/1 -> Divide_0427d/1
  Divide_0427d/1 -> Blockout_d_i_gd_GFL_15_2c157/1

== system IEEE14_case/GFL_15/d_i_gq_GFL_15_block ==
  note: d_i_gq_GFL_15 in case14gfl
      | $\frac{2\,\pi \,\mathrm{Sbase}\,f_{0}\,\left(\Phi _{\mathrm{gd},\mathrm{GFL},15}+P_{\mathrm{iq}}\,\left(\mathrm{Iqv}_{\mathrm{GFL},15}+\Phi _{\mathrm{gc},\mathrm{GFL},15}-i_{\mathrm{gq},\mathrm{GFL},15}-P_{\mathrm{oq}}\,\left(\mathrm{Qe}_{\mathrm{ref}}\,\mathrm{Sbase}+1.73205080756888\,\mathrm{Vbase}\,i_{\mathrm{gd},\mathrm{GFL},15}\,\left(v_{q,\mathrm{GFL},15}\,\cos\left(\theta _{\mathrm{pll},\mathrm{GFL},15}\right)+v_{d,\mathrm{GFL},15}\,\sin\left(\theta _{\mathrm{pll},\mathrm{GFL},15}\right)\right)+1.73205080756888\,\mathrm{Vbase}\,i_{\mathrm{gq},\mathrm{GFL},15}\,\left(v_{d,\mathrm{GFL},15}\,\cos\left(\theta _{\mathrm{pll},\mathrm{GFL},15}\right)-v_{q,\mathrm{GFL},15}\,\sin\left(\theta _{\mathrm{pll},\mathrm{GFL},15}\right)\right)\right)+\mathrm{Bva}\,\mathrm{Vbase}\,\left(v_{q,\mathrm{GFL},15}\,\cos\left(\theta _{\mathrm{pll},\mathrm{GFL},15}\right)+v_{d,\mathrm{GFL},15}\,\sin\left(\theta _{\mathrm{pll},\mathrm{GFL},15}\right)\right)\right)-\frac{\mathrm{Rg}_{\mathrm{pu}}\,{\mathrm{Vbase}}^2\,i_{\mathrm{gq},\mathrm{GFL},15}}{\mathrm{Sbase}}\right)}{\mathrm{Lg}_{\mathrm{pu}}\,{\mathrm{Vbase}}^2}$
      | Automatically generated on 2025-10-09 21:34:56 .
  Input_v_d_GFL_15_d1f59 : Inport
  State_theta_pll_GFL_15_94dd7 : Inport  Port=2
  Input_v_q_GFL_15_1b267 : Inport  Port=3
  State_theta_pll_GFL_15_89960 : Inport  Port=4
  State_Iqv_GFL_15_5d544 : Inport  Port=5
  State_i_gd_GFL_15_18b61 : Inport  Port=6
  Input_v_d_GFL_15_8be69 : Inport  Port=7
  State_theta_pll_GFL_15_b231d : Inport  Port=8
  Input_v_q_GFL_15_75f43 : Inport  Port=9
  State_theta_pll_GFL_15_ed7e5 : Inport  Port=10
  State_i_gq_GFL_15_b1e74 : Inport  Port=11
  Input_v_d_GFL_15_06aad : Inport  Port=12
  State_theta_pll_GFL_15_a894f : Inport  Port=13
  Input_v_q_GFL_15_7f556 : Inport  Port=14
  State_theta_pll_GFL_15_7b0e7 : Inport  Port=15
  State_Phi_gc_GFL_15_ddb2f : Inport  Port=16
  State_i_gq_GFL_15_84adb : Inport  Port=17
  State_Phi_gd_GFL_15_8521d : Inport  Port=18
  State_i_gq_GFL_15_e4e41 : Inport  Port=19
  Add_1a7d6 : Sum
  Add_596a6 : Sum
  Add_774c1 : Sum
  Add_d0f14 : Sum
  Add_f3e39 : Sum
  Add_f61e6 : Sum
  Constant_-1_11a91 : Constant  Value=-1
  Constant_1.73205080756888_6bd8b : Constant  Value=1.73205080756888
  Constant_1.73205080756888_80dd1 : Constant  Value=1.73205080756888
  Constant_2.0_4ffe6 : Constant  Value=2.0
  Constant_2.0_66738 : Constant  Value=2.0
  Constant_2.0_de482 : Constant  Value=2.0
  Constant_Bva_91b2c : Constant  Value=Bva
  Constant_Lg_pu_71b31 : Constant  Value=Lg_pu
  Constant_P_iq_aaaa8 : Constant  Value=P_iq
  Constant_P_oq_a795b : Constant  Value=P_oq
  Constant_Qe_ref_41bbf : Constant  Value=Qe_ref
  Constant_Rg_pu_f426d : Constant  Value=Rg_pu
  Constant_Sbase_4ee8b : Constant  Value=Sbase
  Constant_Sbase_e5ff6 : Constant  Value=Sbase
  Constant_Sbase_fe8b0 : Constant  Value=Sbase
  Constant_Vbase_1c6ef : Constant  Value=Vbase
  Constant_Vbase_291c9 : Constant  Value=Vbase
  Constant_Vbase_92a0d : Constant  Value=Vbase
  Constant_Vbase_e84c8 : Constant  Value=Vbase
  Constant_Vbase_e9ef9 : Constant  Value=Vbase
  Constant_f0_64208 : Constant  Value=f0
  Constant_pi_e9572 : Constant  Value=pi
  Divide_1b972 : Product  Inputs=*/
  Divide_68f64 : Product  Inputs=*/
  MathFunc_cos_1afe5 : Trigonometry  Operator=cos
  MathFunc_cos_2953a : Trigonometry  Operator=cos
  MathFunc_cos_aaa86 : Trigonometry  Operator=cos
  MathFunc_sin_4d565 : Trigonometry
  MathFunc_sin_82866 : Trigonometry
  MathFunc_sin_90323 : Trigonometry
  Power_1238e : Math  Operator=pow
  Power_d3648 : Math  Operator=pow
  Product_03c94 : Product
  Product_06692 : Product
  Product_2da9a : Product
  Product_32fb4 : Product
  Product_35338 : Product
  Product_35fa9 : Product
  Product_4177d : Product
  Product_48338 : Product
  Product_51615 : Product
  Product_5bf32 : Product
  Product_674c9 : Product
  Product_69f4c : Product
  Product_71cc7 : Product
  Product_7ae5f : Product
  Product_824fd : Product
  Product_91c34 : Product
  Product_9e51e : Product
  Product_9fab3 : Product
  Product_a57f1 : Product
  Product_b78c6 : Product
  Product_d2ac3 : Product
  Product_d2d51 : Product
  Product_def5e : Product
  Product_eb774 : Product
  Product_fe17b : Product
  Subtract_00b15 : Sum  Inputs=+-
  Subtract_111cc : Sum  Inputs=+-
  Subtract_245b0 : Sum  Inputs=+-
  Subtract_5cef6 : Sum  Inputs=+-
  Subtract_7b97e : Sum  Inputs=+-
  Blockout_d_i_gq_GFL_15_fa7d1 : Outport
  wires:
  State_theta_pll_GFL_15_b231d/1 -> MathFunc_sin_82866/1
  MathFunc_sin_82866/1 -> Product_2da9a/2
  State_theta_pll_GFL_15_ed7e5/1 -> MathFunc_cos_1afe5/1
  Constant_1.73205080756888_80dd1/1 -> Product_71cc7/1
  MathFunc_cos_1afe5/1 -> Product_b78c6/2
  Product_91c34/1 -> Add_f3e39/1
  Constant_Vbase_e9ef9/1 -> Product_71cc7/2
  State_Iqv_GFL_15_5d544/1 -> Add_d0f14/2
  Input_v_d_GFL_15_8be69/1 -> Product_2da9a/1
  State_i_gq_GFL_15_84adb/1 -> Subtract_00b15/2
  Input_v_q_GFL_15_75f43/1 -> Product_b78c6/1
  State_theta_pll_GFL_15_a894f/1 -> MathFunc_cos_aaa86/1
  State_theta_pll_GFL_15_7b0e7/1 -> MathFunc_sin_90323/1
  Product_5bf32/1 -> Divide_1b972/2
  Constant_Qe_ref_41bbf/1 -> Product_32fb4/2
  State_theta_pll_GFL_15_94dd7/1 -> MathFunc_sin_4d565/1
  State_theta_pll_GFL_15_89960/1 -> MathFunc_cos_2953a/1
  Constant_-1_11a91/1 -> Product_32fb4/1
  Product_71cc7/1 -> Product_fe17b/1
  Subtract_5cef6/1 -> Subtract_7b97e/1
  State_i_gd_GFL_15_18b61/1 -> Product_fe17b/2
  Product_2da9a/1 -> Add_f61e6/1
  Product_b78c6/1 -> Add_f61e6/2
  Constant_1.73205080756888_6bd8b/1 -> Product_9e51e/1
  Constant_2.0_66738/1 -> Power_1238e/2
  Constant_Vbase_1c6ef/1 -> Product_9e51e/2
  Product_674c9/1 -> Product_7ae5f/1
  Constant_Bva_91b2c/1 -> Product_674c9/1
  Add_1a7d6/1 -> Subtract_00b15/1
  Input_v_d_GFL_15_06aad/1 -> Product_eb774/1
  MathFunc_cos_aaa86/1 -> Product_eb774/2
  Product_def5e/1 -> Subtract_245b0/2
  Input_v_q_GFL_15_7f556/1 -> Product_def5e/1
  MathFunc_sin_90323/1 -> Product_def5e/2
  Input_v_d_GFL_15_d1f59/1 -> Product_91c34/1
  Subtract_00b15/1 -> Product_d2ac3/2
  MathFunc_sin_4d565/1 -> Product_91c34/2
  Product_06692/1 -> Add_f3e39/2
  Input_v_q_GFL_15_1b267/1 -> Product_06692/1
  MathFunc_cos_2953a/1 -> Product_06692/2
  Product_32fb4/1 -> Product_35338/1
  Constant_Sbase_e5ff6/1 -> Product_35338/2
  Product_fe17b/1 -> Product_a57f1/1
  Add_f61e6/1 -> Product_a57f1/2
  Product_9e51e/1 -> Product_824fd/1
  Subtract_111cc/1 -> Product_d2d51/2
  State_i_gq_GFL_15_b1e74/1 -> Product_824fd/2
  Product_eb774/1 -> Subtract_245b0/1
  Constant_Vbase_e84c8/1 -> Product_674c9/2
  Product_35338/1 -> Subtract_5cef6/1
  Product_a57f1/1 -> Subtract_5cef6/2
  Constant_2.0_4ffe6/1 -> Product_4177d/1
  Product_824fd/1 -> Product_9fab3/1
  Subtract_245b0/1 -> Product_9fab3/2
  Add_f3e39/1 -> Product_7ae5f/2
  Product_9fab3/1 -> Subtract_7b97e/2
  Power_1238e/1 -> Product_48338/2
  Constant_Vbase_291c9/1 -> Power_1238e/1
  Product_7ae5f/1 -> Add_d0f14/1
  Product_03c94/1 -> Add_596a6/2
  Constant_P_oq_a795b/1 -> Product_03c94/1
  Subtract_7b97e/1 -> Product_03c94/2
  Constant_Rg_pu_f426d/1 -> Product_48338/1
  Constant_f0_64208/1 -> Product_35fa9/2
  Add_d0f14/1 -> Add_596a6/1
  Add_596a6/1 -> Add_1a7d6/1
  State_Phi_gc_GFL_15_ddb2f/1 -> Add_1a7d6/2
  Constant_pi_e9572/1 -> Product_4177d/2
  Constant_P_iq_aaaa8/1 -> Product_d2ac3/1
  Product_48338/1 -> Product_69f4c/1
  Product_d2d51/1 -> Divide_1b972/1
  State_i_gq_GFL_15_e4e41/1 -> Product_69f4c/2
  Product_4177d/1 -> Product_51615/1
  Constant_Sbase_4ee8b/1 -> Product_51615/2
  Product_d2ac3/1 -> Add_774c1/1
  State_Phi_gd_GFL_15_8521d/1 -> Add_774c1/2
  Product_69f4c/1 -> Divide_68f64/1
  Constant_Sbase_fe8b0/1 -> Divide_68f64/2
  Product_51615/1 -> Product_35fa9/1
  Add_774c1/1 -> Subtract_111cc/1
  Divide_68f64/1 -> Subtract_111cc/2
  Constant_Vbase_92a0d/1 -> Power_d3648/1
  Constant_2.0_de482/1 -> Power_d3648/2
  Product_35fa9/1 -> Product_d2d51/1
  Constant_Lg_pu_71b31/1 -> Product_5bf32/1
  Power_d3648/1 -> Product_5bf32/2
  Divide_1b972/1 -> Blockout_d_i_gq_GFL_15_fa7d1/1

== system IEEE14_case/GFL_15/d_theta_pll_GFL_15_block ==
  note: d_theta_pll_GFL_15 in case14gfl
      | $\mathrm{Phipll}_{\mathrm{GFL},15}-P_{\mathrm{pll}}\,\left(\mathrm{vq}_{\mathrm{ref}}+v_{q,\mathrm{GFL},15}\,\cos\left(\theta _{\mathrm{pll},\mathrm{GFL},15}\right)+v_{d,\mathrm{GFL},15}\,\sin\left(\theta _{\mathrm{pll},\mathrm{GFL},15}\right)\right)$
      | Automatically generated on 2025-10-09 21:35:13 .
  Input_v_d_GFL_15_6336d : Inport
  State_theta_pll_GFL_15_a4865 : Inport  Port=2
  Input_v_q_GFL_15_7e43d : Inport  Port=3
  State_theta_pll_GFL_15_f7355 : Inport  Port=4
  State_Phipll_GFL_15_52c7d : Inport  Port=5
  Add_616ef : Sum
  Constant_-1_515d7 : Constant  Value=-1
  Constant_P_pll_ef8a6 : Constant  Value=P_pll
  Constant_vq_ref_fb978 : Constant  Value=vq_ref
  MathFunc_cos_b44c5 : Trigonometry  Operator=cos
  MathFunc_sin_7e942 : Trigonometry
  Product_29412 : Product
  Product_cdaa2 : Product
  Product_e79be : Product
  Product_fc176 : Product
  Subtract_c1d1d : Sum  Inputs=+-
  Subtract_eb8ce : Sum  Inputs=+-
  Blockout_d_theta_pll_GFL_15_bcede : Outport
  wires:
  Input_v_d_GFL_15_6336d/1 -> Product_e79be/2
  Constant_-1_515d7/1 -> Product_e79be/1
  State_theta_pll_GFL_15_a4865/1 -> MathFunc_sin_7e942/1
  State_theta_pll_GFL_15_f7355/1 -> MathFunc_cos_b44c5/1
  MathFunc_cos_b44c5/1 -> Product_29412/2
  Input_v_q_GFL_15_7e43d/1 -> Product_29412/1
  Product_e79be/1 -> Product_fc176/1
  MathFunc_sin_7e942/1 -> Product_fc176/2
  Product_fc176/1 -> Subtract_c1d1d/1
  Product_29412/1 -> Subtract_c1d1d/2
  Subtract_c1d1d/1 -> Subtract_eb8ce/1
  Constant_vq_ref_fb978/1 -> Subtract_eb8ce/2
  State_Phipll_GFL_15_52c7d/1 -> Add_616ef/2
  Constant_P_pll_ef8a6/1 -> Product_cdaa2/1
  Subtract_eb8ce/1 -> Product_cdaa2/2
  Product_cdaa2/1 -> Add_616ef/1
  Add_616ef/1 -> Blockout_d_theta_pll_GFL_15_bcede/1

== system IEEE14_case/GFL_15/e_dc_GFL_15_block ==
  note: e_dc_GFL_15 in case14gfl
      | $\frac{V_{\mathrm{dc},\mathrm{GFL},15}}{\mathrm{Vdcbase}}$
      | Automatically generated on 2025-10-09 21:35:31 .
  State_V_dc_GFL_15_93b67 : Inport
  Constant_Vdcbase_c5f3b : Constant  Value=Vdcbase
  Divide_1ce16 : Product  Inputs=*/
  Blockout_e_dc_GFL_15_d58b9 : Outport
  wires:
  State_V_dc_GFL_15_93b67/1 -> Divide_1ce16/1
  Constant_Vdcbase_c5f3b/1 -> Divide_1ce16/2
  Divide_1ce16/1 -> Blockout_e_dc_GFL_15_d58b9/1

== system IEEE14_case/GFL_15/i_d_GFL_15_block ==
  note: i_d_GFL_15 in case14gfl
      | $0.00658179306876173\,i_{\mathrm{gd},\mathrm{GFL},15}\,\cos\left(\theta _{\mathrm{pll},\mathrm{GFL},15}\right)+0.00658179306876173\,i_{\mathrm{gq},\mathrm{GFL},15}\,\sin\left(\theta _{\mathrm{pll},\mathrm{GFL},15}\right)$
      | Automatically generated on 2025-10-09 21:35:29 .
  State_i_gd_GFL_15_2eb7d : Inport
  State_theta_pll_GFL_15_42e0c : Inport  Port=2
  State_i_gq_GFL_15_49ce8 : Inport  Port=3
  State_theta_pll_GFL_15_0eec4 : Inport  Port=4
  Add_8efe0 : Sum
  Constant_0.00658179306876173_6de94 : Constant  Value=0.00658179306876173
  Constant_0.00658179306876173_79779 : Constant  Value=0.00658179306876173
  MathFunc_cos_41e99 : Trigonometry  Operator=cos
  MathFunc_sin_5807a : Trigonometry
  Product_06cd3 : Product
  Product_7d6e5 : Product
  Product_ccb5a : Product
  Product_f4084 : Product
  Blockout_i_d_GFL_15_9798a : Outport
  wires:
  Constant_0.00658179306876173_6de94/1 -> Product_7d6e5/1
  State_i_gd_GFL_15_2eb7d/1 -> Product_7d6e5/2
  Product_7d6e5/1 -> Product_ccb5a/1
  State_theta_pll_GFL_15_0eec4/1 -> MathFunc_sin_5807a/1
  Product_f4084/1 -> Product_06cd3/1
  State_theta_pll_GFL_15_42e0c/1 -> MathFunc_cos_41e99/1
  Constant_0.00658179306876173_79779/1 -> Product_f4084/1
  MathFunc_cos_41e99/1 -> Product_ccb5a/2
  State_i_gq_GFL_15_49ce8/1 -> Product_f4084/2
  MathFunc_sin_5807a/1 -> Product_06cd3/2
  Product_ccb5a/1 -> Add_8efe0/1
  Product_06cd3/1 -> Add_8efe0/2
  Add_8efe0/1 -> Blockout_i_d_GFL_15_9798a/1

== system IEEE14_case/GFL_15/i_q_GFL_15_block ==
  note: i_q_GFL_15 in case14gfl
      | $0.00658179306876173\,i_{\mathrm{gq},\mathrm{GFL},15}\,\cos\left(\theta _{\mathrm{pll},\mathrm{GFL},15}\right)-0.00658179306876173\,i_{\mathrm{gd},\mathrm{GFL},15}\,\sin\left(\theta _{\mathrm{pll},\mathrm{GFL},15}\right)$
      | Automatically generated on 2025-10-09 21:35:31 .
  State_i_gd_GFL_15_ae75b : Inport
  State_theta_pll_GFL_15_f2c21 : Inport  Port=2
  State_i_gq_GFL_15_dea28 : Inport  Port=3
  State_theta_pll_GFL_15_a18db : Inport  Port=4
  Add_9e943 : Sum
  Constant_-0.00658179306876173_8bf8c : Constant  Value=-0.00658179306876173
  Constant_0.00658179306876173_05e1b : Constant  Value=0.00658179306876173
  MathFunc_cos_acb04 : Trigonometry  Operator=cos
  MathFunc_sin_77d0c : Trigonometry
  Product_0d50a : Product
  Product_628d0 : Product
  Product_d28a9 : Product
  Product_f67db : Product
  Blockout_i_q_GFL_15_86262 : Outport
  wires:
  Add_9e943/1 -> Blockout_i_q_GFL_15_86262/1
  Product_0d50a/1 -> Product_d28a9/1
  Constant_0.00658179306876173_05e1b/1 -> Product_0d50a/1
  Constant_-0.00658179306876173_8bf8c/1 -> Product_628d0/1
  State_theta_pll_GFL_15_f2c21/1 -> MathFunc_sin_77d0c/1
  State_i_gd_GFL_15_ae75b/1 -> Product_628d0/2
  Product_d28a9/1 -> Add_9e943/2
  State_i_gq_GFL_15_dea28/1 -> Product_0d50a/2
  State_theta_pll_GFL_15_a18db/1 -> MathFunc_cos_acb04/1
  MathFunc_sin_77d0c/1 -> Product_f67db/2
  Product_628d0/1 -> Product_f67db/1
  MathFunc_cos_acb04/1 -> Product_d28a9/2
  Product_f67db/1 -> Add_9e943/1

== system IEEE14_case/GFL_16/d_Idv_GFL_16_block ==
  note: d_Idv_GFL_16 in case14gfl
      | $-\frac{\mathrm{Idv}_{\mathrm{GFL},16}+\mathrm{Kdo}\,\left(\mathrm{Vbase}\,\left(v_{q,\mathrm{GFL},16}\,\cos\left(\theta _{\mathrm{pll},\mathrm{GFL},16}\right)+v_{d,\mathrm{GFL},16}\,\sin\left(\theta _{\mathrm{pll},\mathrm{GFL},16}\right)\right)+\frac{\Psi _{d,\mathrm{GFL},16}+\mathrm{Kdi}\,\mathrm{Vbase}\,\left(v_{q,\mathrm{GFL},16}\,\cos\left(\theta _{\mathrm{pll},\mathrm{GFL},16}\right)+v_{d,\mathrm{GFL},16}\,\sin\left(\theta _{\mathrm{pll},\mathrm{GFL},16}\right)\right)}{\mathrm{Tdi}}\right)}{\mathrm{Tdo}}$
      | Automatically generated on 2025-10-09 21:36:18 .
  State_Idv_GFL_16_21a9b : Inport
  Input_v_d_GFL_16_7be83 : Inport  Port=2
  State_theta_pll_GFL_16_5434c : Inport  Port=3
  Input_v_q_GFL_16_b65e9 : Inport  Port=4
  State_theta_pll_GFL_16_fe8ca : Inport  Port=5
  Input_v_d_GFL_16_fb423 : Inport  Port=6
  State_theta_pll_GFL_16_d4b0d : Inport  Port=7
  Input_v_q_GFL_16_07e38 : Inport  Port=8
  State_theta_pll_GFL_16_10000 : Inport  Port=9
  State_Psi_d_GFL_16_8afd7 : Inport  Port=10
  Add_0be75 : Sum
  Add_18da3 : Sum
  Add_76dbc : Sum
  Add_7f093 : Sum
  Constant_-1_2659a : Constant  Value=-1
  Constant_-1_dbb4e : Constant  Value=-1
  Constant_-1_ed55f : Constant  Value=-1
  Constant_Kdi_71269 : Constant  Value=Kdi
  Constant_Kdo_3085b : Constant  Value=Kdo
  Constant_Tdi_9efda : Constant  Value=Tdi
  Constant_Tdo_efa52 : Constant  Value=Tdo
  Constant_Vbase_6849c : Constant  Value=Vbase
  Constant_Vbase_d8930 : Constant  Value=Vbase
  Divide_88984 : Product  Inputs=*/
  Divide_f1415 : Product  Inputs=*/
  MathFunc_cos_2a6bd : Trigonometry  Operator=cos
  MathFunc_cos_e6b26 : Trigonometry  Operator=cos
  MathFunc_sin_9bd7a : Trigonometry
  MathFunc_sin_e4157 : Trigonometry
  Product_56369 : Product
  Product_59828 : Product
  Product_65e28 : Product
  Product_733ec : Product
  Product_7980f : Product
  Product_79c6d : Product
  Product_8b45f : Product
  Product_aa183 : Product
  Product_baded : Product
  Product_c3722 : Product
  Product_d9d87 : Product
  Subtract_7fccb : Sum  Inputs=+-
  Blockout_d_Idv_GFL_16_0d833 : Outport
  wires:
  State_Psi_d_GFL_16_8afd7/1 -> Subtract_7fccb/2
  State_theta_pll_GFL_16_d4b0d/1 -> MathFunc_sin_e4157/1
  State_theta_pll_GFL_16_10000/1 -> MathFunc_cos_e6b26/1
  MathFunc_cos_e6b26/1 -> Product_8b45f/2
  Product_c3722/1 -> Add_0be75/1
  Input_v_d_GFL_16_7be83/1 -> Product_c3722/1
  Constant_Kdi_71269/1 -> Product_aa183/2
  Product_aa183/1 -> Product_59828/1
  Constant_-1_2659a/1 -> Product_aa183/1
  Product_d9d87/1 -> Add_76dbc/1
  Input_v_d_GFL_16_fb423/1 -> Product_d9d87/1
  Constant_Tdo_efa52/1 -> Divide_88984/2
  MathFunc_sin_e4157/1 -> Product_d9d87/2
  Product_8b45f/1 -> Add_76dbc/2
  Input_v_q_GFL_16_07e38/1 -> Product_8b45f/1
  MathFunc_sin_9bd7a/1 -> Product_c3722/2
  State_theta_pll_GFL_16_5434c/1 -> MathFunc_sin_9bd7a/1
  MathFunc_cos_2a6bd/1 -> Product_baded/2
  State_theta_pll_GFL_16_fe8ca/1 -> MathFunc_cos_2a6bd/1
  Constant_Vbase_6849c/1 -> Product_59828/2
  Product_7980f/1 -> Add_7f093/1
  Input_v_q_GFL_16_b65e9/1 -> Product_baded/1
  Constant_-1_ed55f/1 -> Product_7980f/1
  Product_59828/1 -> Product_56369/1
  Add_76dbc/1 -> Product_56369/2
  Constant_-1_dbb4e/1 -> Product_79c6d/1
  Constant_Vbase_d8930/1 -> Product_79c6d/2
  Add_7f093/1 -> Divide_88984/1
  Product_baded/1 -> Add_0be75/2
  Product_56369/1 -> Subtract_7fccb/1
  Product_79c6d/1 -> Product_65e28/1
  Add_0be75/1 -> Product_65e28/2
  Subtract_7fccb/1 -> Divide_f1415/1
  Divide_88984/1 -> Blockout_d_Idv_GFL_16_0d833/1
  Constant_Tdi_9efda/1 -> Divide_f1415/2
  Product_65e28/1 -> Add_18da3/1
  Divide_f1415/1 -> Add_18da3/2
  State_Idv_GFL_16_21a9b/1 -> Product_7980f/2
  Constant_Kdo_3085b/1 -> Product_733ec/1
  Add_18da3/1 -> Product_733ec/2
  Product_733ec/1 -> Add_7f093/2

== system IEEE14_case/GFL_16/d_Iqv_GFL_16_block ==
  note: d_Iqv_GFL_16 in case14gfl
      | $-\frac{\mathrm{Iqv}_{\mathrm{GFL},16}-\mathrm{Kqo}\,\left(\mathrm{Vbase}\,\left(v_{d,\mathrm{GFL},16}\,\cos\left(\theta _{\mathrm{pll},\mathrm{GFL},16}\right)-v_{q,\mathrm{GFL},16}\,\sin\left(\theta _{\mathrm{pll},\mathrm{GFL},16}\right)\right)-\frac{\Psi _{q,\mathrm{GFL},16}-\mathrm{Kqi}\,\mathrm{Vbase}\,\left(v_{d,\mathrm{GFL},16}\,\cos\left(\theta _{\mathrm{pll},\mathrm{GFL},16}\right)-v_{q,\mathrm{GFL},16}\,\sin\left(\theta _{\mathrm{pll},\mathrm{GFL},16}\right)\right)}{\mathrm{Tqi}}\right)}{\mathrm{Tqo}}$
      | Automatically generated on 2025-10-09 21:36:21 .
  State_Iqv_GFL_16_85f35 : Inport
  Input_v_d_GFL_16_a7d3d : Inport  Port=2
  State_theta_pll_GFL_16_74ff7 : Inport  Port=3
  Input_v_q_GFL_16_c2908 : Inport  Port=4
  State_theta_pll_GFL_16_ecda2 : Inport  Port=5
  Input_v_d_GFL_16_3f07a : Inport  Port=6
  State_theta_pll_GFL_16_5893a : Inport  Port=7
  Input_v_q_GFL_16_1ea2b : Inport  Port=8
  State_theta_pll_GFL_16_db814 : Inport  Port=9
  State_Psi_q_GFL_16_4f61f : Inport  Port=10
  Add_00454 : Sum
  Add_19be4 : Sum
  Constant_-1_b7e23 : Constant  Value=-1
  Constant_Kqi_b55c5 : Constant  Value=Kqi
  Constant_Kqo_4a6be : Constant  Value=Kqo
  Constant_Tqi_93910 : Constant  Value=Tqi
  Constant_Tqo_e7c52 : Constant  Value=Tqo
  Constant_Vbase_ab235 : Constant  Value=Vbase
  Constant_Vbase_be8ef : Constant  Value=Vbase
  Divide_138e3 : Product  Inputs=*/
  Divide_1e4c3 : Product  Inputs=*/
  MathFunc_cos_7f994 : Trigonometry  Operator=cos
  MathFunc_cos_f6fd6 : Trigonometry  Operator=cos
  MathFunc_sin_9a9c9 : Trigonometry
  MathFunc_sin_d32ff : Trigonometry
  Product_06af7 : Product
  Product_45606 : Product
  Product_59bdf : Product
  Product_68dd4 : Product
  Product_87e65 : Product
  Product_bc457 : Product
  Product_be01f : Product
  Product_d1001 : Product
  Product_d6080 : Product
  Subtract_228c9 : Sum  Inputs=+-
  Subtract_7354a : Sum  Inputs=+-
  Subtract_76ff7 : Sum  Inputs=+-
  Blockout_d_Iqv_GFL_16_b60c7 : Outport
  wires:
  State_theta_pll_GFL_16_5893a/1 -> MathFunc_cos_7f994/1
  Subtract_228c9/1 -> Product_87e65/2
  MathFunc_sin_9a9c9/1 -> Product_bc457/2
  State_theta_pll_GFL_16_ecda2/1 -> MathFunc_sin_9a9c9/1
  State_theta_pll_GFL_16_db814/1 -> MathFunc_sin_d32ff/1
  Input_v_d_GFL_16_3f07a/1 -> Product_be01f/1
  Product_59bdf/1 -> Add_19be4/1
  MathFunc_cos_7f994/1 -> Product_be01f/2
  Product_d6080/1 -> Subtract_7354a/2
  Input_v_q_GFL_16_1ea2b/1 -> Product_d6080/1
  Constant_-1_b7e23/1 -> Product_59bdf/1
  State_theta_pll_GFL_16_74ff7/1 -> MathFunc_cos_f6fd6/1
  MathFunc_sin_d32ff/1 -> Product_d6080/2
  Product_45606/1 -> Product_68dd4/1
  Constant_Kqi_b55c5/1 -> Product_45606/1
  Constant_Vbase_ab235/1 -> Product_45606/2
  Product_be01f/1 -> Subtract_7354a/1
  Product_d1001/1 -> Subtract_228c9/1
  Input_v_d_GFL_16_a7d3d/1 -> Product_d1001/1
  Subtract_7354a/1 -> Product_68dd4/2
  MathFunc_cos_f6fd6/1 -> Product_d1001/2
  Product_bc457/1 -> Subtract_228c9/2
  Input_v_q_GFL_16_c2908/1 -> Product_bc457/1
  Product_68dd4/1 -> Subtract_76ff7/1
  Product_87e65/1 -> Add_00454/1
  Subtract_76ff7/1 -> Divide_138e3/1
  State_Psi_q_GFL_16_4f61f/1 -> Subtract_76ff7/2
  Constant_Vbase_be8ef/1 -> Product_87e65/1
  Constant_Tqi_93910/1 -> Divide_138e3/2
  Divide_1e4c3/1 -> Blockout_d_Iqv_GFL_16_b60c7/1
  Divide_138e3/1 -> Add_00454/2
  State_Iqv_GFL_16_85f35/1 -> Product_59bdf/2
  Constant_Kqo_4a6be/1 -> Product_06af7/1
  Add_00454/1 -> Product_06af7/2
  Add_19be4/1 -> Divide_1e4c3/1
  Product_06af7/1 -> Add_19be4/2
  Constant_Tqo_e7c52/1 -> Divide_1e4c3/2

== system IEEE14_case/GFL_16/d_Phi_ga_GFL_16_block ==
  note: d_Phi_ga_GFL_16 in case14gfl
      | $I_{\mathrm{od}}\,\left(V_{\mathrm{dc},\mathrm{GFL},16}-\mathrm{Vdcbase}\,\mathrm{Vdc}_{\mathrm{ref}}\right)$
      | Automatically generated on 2025-10-09 21:36:05 .
  State_V_dc_GFL_16_db5ba : Inport
  Constant_I_od_695f0 : Constant  Value=I_od
  Constant_Vdc_ref_02d21 : Constant  Value=Vdc_ref
  Constant_Vdcbase_d2082 : Constant  Value=Vdcbase
  Product_4509e : Product
  Product_863f9 : Product
  Subtract_5d606 : Sum  Inputs=+-
  Blockout_d_Phi_ga_GFL_16_6a1ed : Outport
  wires:
  Product_863f9/1 -> Blockout_d_Phi_ga_GFL_16_6a1ed/1
  Constant_Vdc_ref_02d21/1 -> Product_4509e/1
  Constant_Vdcbase_d2082/1 -> Product_4509e/2
  Product_4509e/1 -> Subtract_5d606/2
  State_V_dc_GFL_16_db5ba/1 -> Subtract_5d606/1
  Constant_I_od_695f0/1 -> Product_863f9/1
  Subtract_5d606/1 -> Product_863f9/2
